simulink model "Station_1_Distributing_Testing"  (R2024a)
settings: Solver=FixedStepAuto  StartTime=0.0  StopTime=30  FixedStep=0.1  RelTol=1e-3
libraries: opcualib x1
settings Model: PacingRate=0.500000  Creator=admin  LastModifiedBy=admin

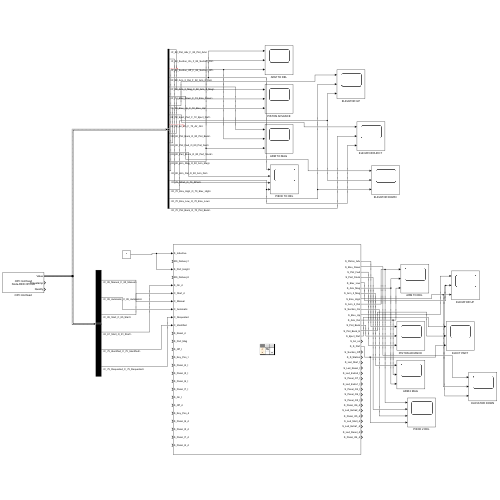
[thumbnail: Simulink's stored preview of the top-level diagram]
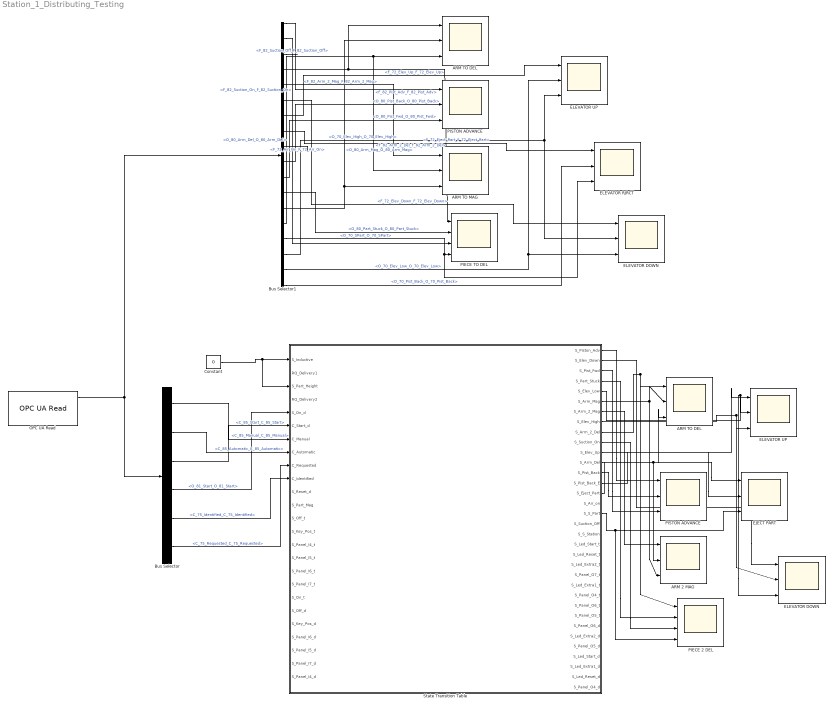
== system Station_1_Distributing_Testing ==
  "ARM 2 MAG " : Scope  NumInputPorts=3
  ARM TO DEL : Scope  NumInputPorts=3
  "ARM TO DEL " : Scope  NumInputPorts=3
  "ARM TO MAG " : Scope  NumInputPorts=3
  Bus Selector : BusSelector  OutputSignals=C_85_Manual_C_85_Manual,C_85_Automatic_C_85_Automatic,C_85_Start_C_85_Start,O_81_Start_O_81_Start,C_75_Identified_C_75_Identified,C_75_Requested_C_75_Requested
  Bus Selector1 : BusSelector  OutputSignals=F_82_Pist_Adv_F_82_Pist_Adv,F_82_Suction_On_F_82_Suction_On,F_82_Suction_Off_F_82_Suction_Off,F_82_Arm_2_Del_F_82_Arm_2_Del,F_82_Arm_2_Mag_F_82_Arm_2_Mag,F_72_Elev_Down_F_72_Elev_Down,F_72_Elev_Up_F_72_Elev_Up,F_72_Eject_Part_F_72_Eject_Part,F_72_Air_On_F_72_Air_On,O_80_Pist_Back_O_80_Pist_Back,O_80_Pist_Fwd_O_80_Pist_Fwd,O_80_Part_Stuck_O_80_Part_Stuck,O_80_Arm_Mag_O_80_Arm_Mag,O_80_Arm_Del_O_80_Arm_Del,O_70_SPart_O_70_SPart,O_70_Elev_High_O_70_Elev_High,O_70_Elev_Low_O_70_Elev_Low,O_70_Pist_Back_O_70_Pist_Back
  Constant : Constant  Value=0
  EJECT PART : Scope  NumInputPorts=3
  ELEVATOR DOWN : Scope  NumInputPorts=3
  "ELEVATOR DOWN " : Scope  NumInputPorts=3
  "ELEVATOR RJRCT " : Scope  NumInputPorts=3
  ELEVATOR UP : Scope  NumInputPorts=3
  "ELEVATOR UP " : Scope  NumInputPorts=3
  OPC UA Read : opcualib/OPC UA Read  SelectedServer=Node-RED OPCUA  ServerList=Node-RED OPCUA  NodeList={ '1', 'C_85_Manual', '17', 'C_85_Manual', '0'; '2', 'C_85_Automatic', '17', 'C_85_Automatic', '0'; '3', 'C_85_Start', '17', 'C_85_Start', '0'; '4', 'O_81_Start', '17', 'O_81_Start', '0'; '5', 'F_82_Pist_Adv', '17', 'F_82_Pist_Adv', '0'; '6', 'F_82_Suction_On', '17', 'F_82_Suction_On', '0'; '7', 'F_82_Suction_Off', '17', 'F_82_Suction_Off', '0'; '8', 'F_82_Arm_2_Del', '17', 'F_82_Arm_2_Del', '0'; '9', 'F_82_Arm_2_Mag', '17', 'F_82_Arm_2_Mag', '0'; '10', 'F_72_Elev_Down', '16', 'F_72_Elev_Down', '0'; '11', 'F_72_Elev_Up', '16', 'F_72_Elev_Up', '0'; '12', 'F_72_Eject_Part', '16', 'F_72_Eject_Part', '0'; '13', 'F_72_Air_On', '16', 'F_72_Air_On', '0'; '14', 'C_75_Identified', '16', 'C_75_Identified', '0'; '15', 'C_75_Requested', '16', 'C_75_Requested', '0'; '16', 'O_80_Pist_Back', '17', 'O_80_Pist_Back', '0'; '17', 'O_80_Pist_Fwd', '17', 'O_80_Pist_Fwd', '0'; '18', 'O_80_Part_Stuck', '17', 'O_80_Part_Stuck', '0'; '19', 'O_80_Arm_Mag', '17', 'O_80_Arm_Mag', '0'; '20', 'O_80_Arm_Del', '17', 'O_80_Arm_Del', '0'; '21', 'O_70_SPart', '16', 'O_70_SPart', '0'; '22', 'O_70_Elev_High', '16', 'O_70_Elev_High', '0'; '23', 'O_70_Elev_Low', '16', 'O_70_Elev_Low', '0'; '24', 'O_70_Pist_Back', '16', 'O_70_Pist_Back', '0' }  ShowQualityPort=on  ShowTimestampPort=on  ShowTimestampPortAs=Seconds since start  SampleTime=-1
  PIECE 2 DEL : Scope  NumInputPorts=4
  PIECE TO DEL : Scope  NumInputPorts=4
  PISTON ADVANCE : Scope  NumInputPorts=3
  "PISTON ADVANCE " : Scope  NumInputPorts=3
  State Transition Table : State Transition Table  TreatAsAtomicUnit=on
      settings: PortSchema="{\"entries\":[{\"content\":{\"sides\":[{\"content\":{\"connectorIds\":[\"In1\",\"In2\",\"In3\",\"In4\",\"In5\",\"In6\",\"In7\",\"In8\",\"In9\",\"In10\",\"In11\",\"In12\",\"In13\",\"In14\",\"In15\",\"In16\",\"In17\",\"In18\",\"In19\",\"In20\",\"In21\",\"In22\",\"In23\",\"In24\",\"In25\"]},\"type\":\"ConnectorPlacement.EquallySpacedRectSide\",\"uuid\":\"c1ffde1c-4698-47c1-b8e1-e37e2294cce5\"},{\"content\":{\"connectorIds\":[\"Out1\",\"Out2\",\"Out3\",\"Out4\",\"Out5\",\"Out6\",\"Out7\",\"Out8\",\"Out10\",\"Out9\",\"Out11\",\"Out12\",\"Out13\",\"Out14\",\"Out15\",\"Out16\",\"Out17\",\"Out18\",\"Out19\",\"Out20\",\"Out21\",\"Out22\",\"Out23\",\"Out24\",\"Out25\",\"Out26\",\"Out27\",\"Out28\",\"Out29\",\"Out30\",\"Out31\",\"Out32\",\"Out33\",\"Out34\"],\"side\":\"RIGHT\"},\"type\":\"ConnectorPlacement.EquallySpacedRectSide\",\"uuid\":\"c7cc1e75-ba3b-429d-be47-1a37eca50664\"},{\"content\":{\"side\":\"TOP\"},\"type\":\"ConnectorPlacement.EquallySpacedRectSide\",\"uuid\":\"a3e10976-981e-41c1-9e4c-ac87463bc268\"}]},\"type\":\"ConnectorPlacement.EquallySpacedConnector\",\"uuid\":\"49dd4243-5969-4559-99a9-f798051ededc\"}],\"packageUris\":[\"http://schema.mathworks.com/mf0/Connector/R2020b\"],\"version\":\"1.0\"}"
  wires:
  OPC UA Read/1 -> Bus Selector/1, Bus Selector1/1
  Bus Selector/1 -> State Transition Table/7(C_Manual)  "<C_85_Manual_C_85_Manual>"
  Bus Selector/2 -> State Transition Table/8(C_Automatic)  "<C_85_Automatic_C_85_Automatic>"
  Bus Selector/4 -> State Transition Table/5(S_On_d)  "<O_81_Start_O_81_Start>"
  Bus Selector/3 -> State Transition Table/6(C_Start_d)  "<C_85_Start_C_85_Start>"
  Constant/1 -> State Transition Table/1(S_Inductive), State Transition Table/3(S_Part_Height)
  Bus Selector/5 -> State Transition Table/10(C_Identified)  "<C_75_Identified_C_75_Identified>"
  Bus Selector/6 -> State Transition Table/9(C_Requested)  "<C_75_Requested_C_75_Requested>"
  Bus Selector1/1 -> PISTON ADVANCE/1  "<F_82_Pist_Adv_F_82_Pist_Adv>"
  Bus Selector1/2 -> PIECE TO DEL/3  "<F_82_Suction_On_F_82_Suction_On>"
  Bus Selector1/3 -> ?  "<F_82_Suction_Off_F_82_Suction_Off>"
  Bus Selector1/4 -> PIECE TO DEL/1, ARM TO DEL/1  "<F_82_Arm_2_Del_F_82_Arm_2_Del>"
  Bus Selector1/5 -> "ARM TO MAG "/1  "<F_82_Arm_2_Mag_F_82_Arm_2_Mag>"
  Bus Selector1/6 -> "ELEVATOR DOWN "/1  "<F_72_Elev_Down_F_72_Elev_Down>"
  Bus Selector1/7 -> ELEVATOR UP/1  "<F_72_Elev_Up_F_72_Elev_Up>"
  Bus Selector1/8 -> "ELEVATOR RJRCT "/1  "<F_72_Eject_Part_F_72_Eject_Part>"
  Bus Selector1/9 -> ?  "<F_72_Air_On_F_72_Air_On>"
  Bus Selector1/10 -> PISTON ADVANCE/2  "<O_80_Pist_Back_O_80_Pist_Back>"
  Bus Selector1/11 -> PISTON ADVANCE/3  "<O_80_Pist_Fwd_O_80_Pist_Fwd>"
  Bus Selector1/13 -> "ARM TO MAG "/3, ARM TO DEL/2  "<O_80_Arm_Mag_O_80_Arm_Mag>"
  Bus Selector1/14 -> ARM TO DEL/3, "ARM TO MAG "/2  "<O_80_Arm_Del_O_80_Arm_Del>"
  Bus Selector1/15 -> "ELEVATOR RJRCT "/3, PIECE TO DEL/4  "<O_70_SPart_O_70_SPart>"
  Bus Selector1/16 -> "ELEVATOR DOWN "/2, ELEVATOR UP/3  "<O_70_Elev_High_O_70_Elev_High>"
  Bus Selector1/17 -> "ELEVATOR DOWN "/3, ELEVATOR UP/2  "<O_70_Elev_Low_O_70_Elev_Low>"
  Bus Selector1/18 -> "ELEVATOR RJRCT "/2  "<O_70_Pist_Back_O_70_Pist_Back>"
  Bus Selector1/12 -> PIECE TO DEL/2  "<O_80_Part_Stuck_O_80_Part_Stuck>"
  State Transition Table/10(S_Arm_2_Del) -> PIECE 2 DEL/1, "ARM TO DEL "/1
  State Transition Table/6(S_Arm_Mag) -> "ARM 2 MAG "/3, "ARM TO DEL "/2
  State Transition Table/12(S_Arm_Del) -> "ARM 2 MAG "/2, "ARM TO DEL "/3
  State Transition Table/1(S_Piston_Adv) -> "PISTON ADVANCE "/1
  State Transition Table/13(S_Pist_Back) -> "PISTON ADVANCE "/2
  State Transition Table/3(S_Pist_Fwd) -> "PISTON ADVANCE "/3
  State Transition Table/7(S_Arm_2_Mag) -> "ARM 2 MAG "/1
  State Transition Table/4(S_Part_Stuck) -> PIECE 2 DEL/2
  State Transition Table/9(S_Suction_On) -> PIECE 2 DEL/3
  State Transition Table/11(S_Elev_Up) -> "ELEVATOR UP "/1
  State Transition Table/5(S_Elev_Low) -> ELEVATOR DOWN/3, "ELEVATOR UP "/2
  State Transition Table/8(S_Elev_High) -> ELEVATOR DOWN/2, "ELEVATOR UP "/3
  State Transition Table/15(S_Eject_Part) -> EJECT PART/1
  State Transition Table/14(S_Pist_Back_E) -> EJECT PART/2
  State Transition Table/17(S_S_Part) -> PIECE 2 DEL/4, EJECT PART/3
  State Transition Table/2(S_Elev_Down) -> ELEVATOR DOWN/1

== stateflow chart Station_1_Distributing_Testing/State Transition Table ==
  state state1
    S_Arm_2_Del=0;
    S_Arm_2_Mag=0;
    S_Piston_Adv=0;
    S_Elev_Up=0;
    S_Elev_Down=0;
    S_Eject_Part=0;
    S_Air_on=0;
    S_Suction_On=0;
    S_Suction_Off=0;
    S_Arm_Mag=1;
    S_Arm_Del=0;
    S_Part_Stuck=0;
    S_Pist_Fwd=0;
    S_Pist_Back=1;
    S_Elev_Low=1;
    S_Elev_High=0;
    S_S_Part=0;
    S_Pist_Back_E=1;
    S_S_Station=0;
    S_On_t;
    S_Off_t;
    S_Key_Pos_t;
    S_Panel_I4_t;
    S_Panel_I5_t;
    S_Panel_I6_t;
    S_Panel_I7_t;
    S_Led_Start_t=0;
    S_Led_Reset_t=0;
    S_Led_Extra1_t=0;
    S_Led_Extra2_t=0;
    S_Panel_O4_t=0;
    S_Panel_O5_t=0;
    S_Panel_O6_t=0;
    S_Panel_O7_t=0;
    S_Off_d;
    S_Key_Pos_d;
    S_Panel_I4_d;
    S_Panel_I5_d;
    S_Panel_I6_d;
    S_Panel_I7_d;
    S_Led_Start_d=0;
    S_Led_Reset_d=0;
    S_Led_Extra1_d=0;
    S_Led_Extra2_d=0;
    S_Panel_O4_d=0;
    S_Panel_O5_d=0;
    S_Panel_O6_d=0;
  state dis_cont_arm_to_del
    S_Arm_2_Del=1;
    S_Arm_2_Mag=0;
    S_Piston_Adv=0;
    S_Elev_Up=0;
    S_Elev_Down=0;
    S_Eject_Part=0;
    S_Air_on=0;
    S_Suction_On=0;
    state dis_cont_arm_to_del_1
    (default) -> dis_cont_arm_to_del_1
    dis_cont_arm_to_del_1 -> (junction 261) : after(0.73,sec)
        | {S_Arm_Mag=0;}
    (junction 261) -> dis_cont_arm_to_del_1
  state piston_advance
    S_Arm_2_Del=0;
    S_Arm_2_Mag=0;
    S_Piston_Adv=1;
    S_Elev_Up=0;
    S_Elev_Down=0;
    S_Eject_Part=0;
    S_Air_on=0;
    S_Suction_On=0;
    state piston_advance_1
    (default) -> piston_advance_1
    piston_advance_1 -> (junction 257) : {S_Pist_Back=0;
        | S_Pist_Fwd=1;}
    (junction 257) -> piston_advance_1
  state arm_to_mag
    S_Arm_2_Del=0;
    S_Arm_2_Mag=1;
    S_Piston_Adv=0;
    S_Elev_Up=0;
    S_Elev_Down=0;
    S_Eject_Part=0;
    S_Air_on=0;
    S_Suction_On=0;
    state arm_to_mag_1
    (default) -> arm_to_mag_1
    arm_to_mag_1 -> (junction 269) : after(0.5,sec)
        | {S_Arm_Del=0;}
    (junction 269) -> arm_to_mag_1
  state arm_with_piece_to_del
    S_Arm_2_Del=1;
    S_Arm_2_Mag=0;
    S_Piston_Adv=0;
    S_Elev_Up=0;
    S_Elev_Down=0;
    S_Eject_Part=0;
    S_Air_on=0;
    S_Suction_On=1;
    state arm_with_piece_to_del_1
    (default) -> arm_with_piece_to_del_1
    arm_with_piece_to_del_1 -> (junction 265) : after(0.73,sec)
        | {S_Arm_Mag=0;}
    (junction 265) -> arm_with_piece_to_del_1
  state arm_to_mag1
    S_Arm_2_Del=0;
    S_Arm_2_Mag=1;
    S_Piston_Adv=0;
    S_Elev_Up=0;
    S_Elev_Down=0;
    S_Eject_Part=0;
    S_Air_on=0;
    S_Suction_On=0;
    state arm_to_mag1_1
    state arm_to_mag1_2
    arm_to_mag1_2 -> (junction 974) : after(0.2,sec)
        | {S_Arm_Del=0;}
    (default) -> arm_to_mag1_1
    arm_to_mag1_1 -> arm_to_mag1_2 : [after(0.5,sec)]
        | {S_Suction_Off=0;}
    (junction 974) -> arm_to_mag1_2
  state elevator_up
    S_Arm_2_Del=0;
    S_Arm_2_Mag=0;
    S_Piston_Adv=0;
    S_Elev_Up=1;
    S_Elev_Down=0;
    S_Eject_Part=0;
    S_Air_on=0;
    S_Suction_On=0;
    state elevator_up_1
    state elevator_up_2
    state elevator_up_3
    state elevator_up_4
    elevator_up_4 -> (junction 1045) : after(0.65,sec)
        | {S_Elev_High=1;}
    (default) -> elevator_up_1
    elevator_up_1 -> elevator_up_2 : after(0.5,sec)
        | {S_Elev_Low=0;}
    elevator_up_2 -> elevator_up_3 : after(0.1,sec)
        | {S_S_Station=1;}
    elevator_up_3 -> elevator_up_4 : after(0.3,sec)
        | {S_S_Station=1;}
    (junction 1045) -> elevator_up_4
  state decision
  state accepted
    S_Arm_2_Del=0;
    S_Arm_2_Mag=0;
    S_Piston_Adv=0;
    S_Elev_Up=1;
    S_Elev_Down=0;
    S_Eject_Part=1;
    S_Air_on=1;
    S_Suction_On=0;
    state accepted_1
    (default) -> accepted_1
    accepted_1 -> (junction 291) : after(0.2,sec)
        | {S_Pist_Back_E=0;}
    (junction 291) -> accepted_1
  state elevator_down
    S_Arm_2_Del=0;
    S_Arm_2_Mag=0;
    S_Piston_Adv=0;
    S_Elev_Up=0;
    S_Elev_Down=1;
    S_Eject_Part=0;
    S_Air_on=1;
    S_Suction_On=0;
    state elevator_down_1
    state elevator_down_2
    state elevator_down_3
    state elevator_down_4
    elevator_down_4 -> (junction 987) : after(0.3,sec)
        | {S_S_Station=0;}
    (default) -> elevator_down_1
    elevator_down_1 -> elevator_down_2 : after(0.2,sec)
        | {S_Pist_Back_E=1;}
    elevator_down_2 -> elevator_down_3 : after(0.1,sec)
        | {S_Elev_High=0;}
    elevator_down_3 -> elevator_down_4 : after(0.7,sec)
        | {S_S_Station=1;}
    (junction 987) -> elevator_down_4
  state elev_is_down_but_air
    S_Arm_2_Del=0;
    S_Arm_2_Mag=0;
    S_Piston_Adv=0;
    S_Elev_Up=0;
    S_Elev_Down=0;
    S_Eject_Part=0;
    S_Air_on=1;
    S_Suction_On=0;
  state rejected
    S_Arm_2_Del=0;
    S_Arm_2_Mag=0;
    S_Piston_Adv=0;
    S_Elev_Up=0;
    S_Elev_Down=1;
    S_Eject_Part=0;
    S_Air_on=0;
    S_Suction_On=0;
    state rejected_1
    state rejected_2
    state rejected_3
    rejected_3 -> (junction 993) : after(0.3,sec)
        | {S_S_Station=0;}
    (default) -> rejected_1
    rejected_1 -> rejected_2 : after(0.3,sec)
        | {S_Elev_High=0;}
    rejected_2 -> rejected_3 : after(0.7,sec)
        | {S_S_Station=1;}
    (junction 993) -> rejected_3
  state rejection_ejection
    S_Arm_2_Del=0;
    S_Arm_2_Mag=0;
    S_Piston_Adv=0;
    S_Elev_Up=0;
    S_Elev_Down=0;
    S_Eject_Part=1;
    S_Air_on=0;
    S_Suction_On=0;
    state rejection_ejection_1
    (default) -> rejection_ejection_1
    rejection_ejection_1 -> (junction 305) : after(0.2,sec)
        | {S_Pist_Back_E=0;}
    (junction 305) -> rejection_ejection_1
  state pistonback
  state cont_arm_to_delivery
    S_Arm_2_Del=1;
    S_Arm_2_Mag=0;
    S_Piston_Adv=0;
    S_Elev_Up=0;
    S_Elev_Down=0;
    S_Eject_Part=0;
    S_Air_on=0;
    S_Suction_On=0;
    state cont_arm_to_delivery_1
    (default) -> cont_arm_to_delivery_1
    cont_arm_to_delivery_1 -> (junction 317) : after(0.73,sec)
        | {S_Arm_Mag=0;}
    (junction 317) -> cont_arm_to_delivery_1
  state arm_to_delivery_pist_adv
    S_Arm_2_Del=1;
    S_Arm_2_Mag=0;
    S_Piston_Adv=1;
    S_Elev_Up=0;
    S_Elev_Down=0;
    S_Eject_Part=0;
    S_Air_on=0;
    S_Suction_On=0;
    state arm_to_delivery_pist_adv_1
    (default) -> arm_to_delivery_pist_adv_1
    arm_to_delivery_pist_adv_1 -> (junction 555) : {S_Pist_Fwd=1;
        | S_Pist_Back=0;}
    (junction 555) -> arm_to_delivery_pist_adv_1
  state arm_to_mag_cont
    S_Arm_2_Del=0;
    S_Arm_2_Mag=1;
    S_Piston_Adv=0;
    S_Elev_Up=0;
    S_Elev_Down=0;
    S_Eject_Part=0;
    S_Air_on=0;
    S_Suction_On=0;
    state arm_to_mag_cont_1
    (default) -> arm_to_mag_cont_1
    arm_to_mag_cont_1 -> (junction 324) : after(0.73,sec)
        | {S_Arm_Del=0;}
    (junction 324) -> arm_to_mag_cont_1
  state piece_to_del1
    S_Arm_2_Del=1;
    S_Arm_2_Mag=0;
    S_Piston_Adv=0;
    S_Elev_Up=0;
    S_Elev_Down=0;
    S_Eject_Part=0;
    S_Air_on=0;
    S_Suction_On=1;
    state piece_to_del1_1
    (default) -> piece_to_del1_1
    piece_to_del1_1 -> (junction 396) : after(0.73,sec)
        | {S_Arm_Mag=0;}
    (junction 396) -> piece_to_del1_1
  state piece_to_del2
    S_Arm_2_Del=1;
    S_Arm_2_Mag=0;
    S_Piston_Adv=0;
    S_Elev_Up=0;
    S_Elev_Down=0;
    S_Eject_Part=0;
    S_Air_on=0;
    S_Suction_On=1;
  state arm_to_mag_pist_adv
    S_Arm_2_Del=0;
    S_Arm_2_Mag=1;
    S_Piston_Adv=1;
    S_Elev_Up=0;
    S_Elev_Down=0;
    S_Eject_Part=0;
    S_Air_on=0;
    S_Suction_On=0;
    state arm_to_mag_pist_adv_1
    state arm_to_mag_pist_adv_2
    arm_to_mag_pist_adv_2 -> (junction 997) : after(0.3,sec)
        | {S_Suction_Off=0;}
    (default) -> arm_to_mag_pist_adv_1
    arm_to_mag_pist_adv_1 -> arm_to_mag_pist_adv_2 : after(0.2,sec)
        | {S_S_Part=1;}
    (junction 997) -> arm_to_mag_pist_adv_2
  state rest_of_arm_to_mag
    S_Arm_2_Del=0;
    S_Arm_2_Mag=1;
    S_Piston_Adv=0;
    S_Elev_Up=0;
    S_Elev_Down=0;
    S_Eject_Part=0;
    S_Air_on=0;
    S_Suction_On=0;
    state rest_of_arm_to_mag_1
    (default) -> rest_of_arm_to_mag_1
    rest_of_arm_to_mag_1 -> (junction 410) : after(0.13,sec)
        | {S_Arm_Del=0;}
    (junction 410) -> rest_of_arm_to_mag_1
  state elevtor_up_cont
    S_Arm_2_Del=0;
    S_Arm_2_Mag=0;
    S_Piston_Adv=0;
    S_Elev_Up=1;
    S_Elev_Down=0;
    S_Eject_Part=0;
    S_Air_on=0;
    S_Suction_On=1;
    S_Part_Stuck=1;
    state elevtor_up_cont_1
    state elevtor_up_cont_2
    state elevtor_up_cont_3
    state elevtor_up_cont_4
    elevtor_up_cont_4 -> (junction 1005) : after(0.65,sec)
        | {S_Elev_High=1;}
    (default) -> elevtor_up_cont_1
    elevtor_up_cont_1 -> elevtor_up_cont_2 : after(0.50,sec)
        | {S_Elev_Low=0;}
    elevtor_up_cont_2 -> elevtor_up_cont_3 : after(0.1,sec)
        | {S_S_Station=1;}
    elevtor_up_cont_3 -> elevtor_up_cont_4 : after(0.3,sec)
        | {S_S_Station=0;}
    (junction 1005) -> elevtor_up_cont_4
  state decicion_2
  state accept2
    S_Arm_2_Del=0;
    S_Arm_2_Mag=0;
    S_Piston_Adv=0;
    S_Elev_Up=1;
    S_Elev_Down=0;
    S_Eject_Part=1;
    S_Air_on=1;
    S_Suction_On=1;
    state accept2_1
    (default) -> accept2_1
    accept2_1 -> (junction 571) : after(0.2,sec)
        | {S_Pist_Back_E=0;}
    (junction 571) -> accept2_1
  state elevator_down2
    S_Arm_2_Del=0;
    S_Arm_2_Mag=0;
    S_Piston_Adv=0;
    S_Elev_Up=0;
    S_Elev_Down=1;
    S_Eject_Part=0;
    S_Air_on=1;
    S_Suction_On=1;
    state elevator_down2_1
      state elevator_down2_1_1
        state elevator_down2_1_1_1
        (default) -> elevator_down2_1_1_1
        elevator_down2_1_1_1 -> (junction 848) : after(0.3,sec)
            | {S_Elev_High=0;}
        (junction 848) -> elevator_down2_1_1_1
      (default) -> elevator_down2_1_1
      elevator_down2_1_1 -> (junction 443) : after(1,sec)
          | {S_S_Station=1;}
      (junction 443) -> elevator_down2_1_1
    (default) -> elevator_down2_1
    elevator_down2_1 -> (junction 439) : after(1.3,sec)
        | {S_S_Station=0;}
    (junction 439) -> elevator_down2_1
  state to_del2_1
    S_Arm_2_Del=1;
    S_Arm_2_Mag=0;
    S_Piston_Adv=0;
    S_Elev_Up=0;
    S_Elev_Down=0;
    S_Eject_Part=0;
    S_Air_on=1;
    S_Suction_On=1;
    state to_del2_1_1
    (default) -> to_del2_1_1
    to_del2_1_1 -> (junction 575) : after(0.73,sec)
        | {S_Arm_Mag=0;}
    (junction 575) -> to_del2_1_1
  state reject2
    S_Arm_2_Del=0;
    S_Arm_2_Mag=0;
    S_Piston_Adv=0;
    S_Elev_Up=0;
    S_Elev_Down=1;
    S_Eject_Part=0;
    S_Air_on=0;
    S_Suction_On=1;
    state reject2_1
    state reject2_2
    state reject2_3
    reject2_3 -> (junction 1012) : after(0.3,sec)
        | {S_S_Station=0;}
    (default) -> reject2_1
    reject2_1 -> reject2_2 : after(0.3,sec)
        | {S_Elev_High=0;}
    reject2_2 -> reject2_3 : after(0.7,sec)
        | {S_S_Station=1;}
    (junction 1012) -> reject2_3
  state arm_to_del_with_eject
    S_Arm_2_Del=1;
    S_Arm_2_Mag=0;
    S_Piston_Adv=0;
    S_Elev_Up=0;
    S_Elev_Down=0;
    S_Eject_Part=1;
    S_Air_on=0;
    S_Suction_On=1;
    state arm_to_del_with_eject_1
    state arm_to_del_with_eject_2
    arm_to_del_with_eject_2 -> (junction 1020) : after(0.5,sec)
        | {S_Arm_Mag=0;}
    (default) -> arm_to_del_with_eject_1
    arm_to_del_with_eject_1 -> arm_to_del_with_eject_2 : after(0.2,sec)
        | {S_Pist_Back_E=0;}
    (junction 1020) -> arm_to_del_with_eject_2
  state after_last_piece_delivery
    S_Arm_2_Del=0;
    S_Arm_2_Mag=1;
    S_Piston_Adv=0;
    S_Elev_Up=0;
    S_Elev_Down=0;
    S_Eject_Part=0;
    S_Air_on=0;
    S_Suction_On=0;
    state after_last_piece_delivery_1
    state after_last_piece_delivery_2
    after_last_piece_delivery_2 -> (junction 1016) : after(0.50,sec)
        | {S_Arm_Del=0;}
    (default) -> after_last_piece_delivery_1
    after_last_piece_delivery_1 -> after_last_piece_delivery_2 : after(0.2,sec)
        | {S_S_Part=1;}
    (junction 1016) -> after_last_piece_delivery_2
  state elevator_up_with_to_mag
    S_Arm_2_Del=0;
    S_Arm_2_Mag=1;
    S_Piston_Adv=0;
    S_Elev_Up=1;
    S_Elev_Down=0;
    S_Eject_Part=0;
    S_Air_on=0;
    S_Suction_On=0;
  state elevator_up_only
    S_Arm_2_Del=0;
    S_Arm_2_Mag=1;
    S_Piston_Adv=0;
    S_Elev_Up=1;
    S_Elev_Down=0;
    S_Eject_Part=0;
    S_Air_on=0;
    S_Suction_On=0;
    state elevator_up_only_1
    state elevator_up_only_2
    state elevator_up_only_3
    state elevator_up_only_4
    elevator_up_only_4 -> (junction 1028) : after(0.65,sec)
        | {S_Elev_High=1;}
    (default) -> elevator_up_only_1
    elevator_up_only_1 -> elevator_up_only_2 : after(0.3,sec)
        | {S_Elev_Low=0;}
    elevator_up_only_2 -> elevator_up_only_3 : after(0.1,sec)
        | {S_S_Station=1;}
    elevator_up_only_3 -> elevator_up_only_4 : after(0.3,sec)
        | {S_S_Station=0;}
    (junction 1028) -> elevator_up_only_4
  state decision_3
  state accept
    S_Arm_2_Del=0;
    S_Arm_2_Mag=0;
    S_Piston_Adv=0;
    S_Elev_Up=1;
    S_Elev_Down=0;
    S_Eject_Part=1;
    S_Air_on=1;
    S_Suction_On=0;
  state elev_down_4
    S_Arm_2_Del=0;
    S_Arm_2_Mag=0;
    S_Piston_Adv=0;
    S_Elev_Up=0;
    S_Elev_Down=1;
    S_Eject_Part=0;
    S_Air_on=1;
    S_Suction_On=0;
    state elev_down_4_1
    state elev_down_4_2
    state elev_down_4_3
    state elev_down_4_4
    elev_down_4_4 -> (junction 1036) : after(0.3,sec)
        | {S_S_Station=0;}
    (default) -> elev_down_4_1
    elev_down_4_1 -> elev_down_4_2 : after(0.2,sec)
        | {S_Pist_Back_E=1;}
    elev_down_4_2 -> elev_down_4_3 : after(0.1,sec)
        | {S_Elev_High=0;}
    elev_down_4_3 -> elev_down_4_4 : after(0.7,sec)
        | {S_S_Station=1;}
    (junction 1036) -> elev_down_4_4
  state air_still_on
    S_Arm_2_Del=0;
    S_Arm_2_Mag=0;
    S_Piston_Adv=0;
    S_Elev_Up=0;
    S_Elev_Down=0;
    S_Eject_Part=0;
    S_Air_on=1;
    S_Suction_On=0;
  state reject_elev_down
    S_Arm_2_Del=0;
    S_Arm_2_Mag=0;
    S_Piston_Adv=0;
    S_Elev_Up=0;
    S_Elev_Down=1;
    S_Eject_Part=0;
    S_Air_on=0;
    S_Suction_On=0;
    state reject_elev_down_1
    state reject_elev_down_2
    state reject_elev_down_3
    reject_elev_down_3 -> (junction 1042) : after(0.3,sec)
        | {S_S_Station=0;}
    (default) -> reject_elev_down_1
    reject_elev_down_1 -> reject_elev_down_2 : after(0.3,sec)
        | {S_Elev_High=0;}
    reject_elev_down_2 -> reject_elev_down_3 : after(0.7,sec)
        | {S_S_Station=1;}
    (junction 1042) -> reject_elev_down_3
  state ejecting_part
    S_Arm_2_Del=0;
    S_Arm_2_Mag=0;
    S_Piston_Adv=0;
    S_Elev_Up=0;
    S_Elev_Down=0;
    S_Eject_Part=1;
    S_Air_on=0;
    S_Suction_On=0;
    state ejecting_part_1
    (default) -> ejecting_part_1
    ejecting_part_1 -> (junction 583) : after(0.2,sec)
        | {S_Pist_Back_E=0;}
    (junction 583) -> ejecting_part_1
  state piston_back_sensor
  state RESET
    S_Arm_2_Del=0;
    S_Arm_2_Mag=0;
    S_Piston_Adv=0;
    S_Elev_Up=0;
    S_Elev_Down=0;
    S_Eject_Part=0;
    S_Air_on=0;
    S_Suction_On=0;
    S_Suction_Off=0;
  state reset_RETURN_ARM_TO_MAG_with_suction
    S_Arm_2_Del=0;
    S_Arm_2_Mag=1;
    S_Piston_Adv=0;
    S_Elev_Up=0;
    S_Elev_Down=0;
    S_Eject_Part=0;
    S_Air_on=0;
    S_Suction_On=1;
    S_Suction_Off=0;
  state suction_off_reset
    S_Arm_2_Del=0;
    S_Arm_2_Mag=0;
    S_Piston_Adv=0;
    S_Elev_Up=0;
    S_Elev_Down=0;
    S_Eject_Part=0;
    S_Air_on=0;
    S_Suction_On=0;
    S_Suction_Off=1;
  state reset_return_arm_to_mag
    S_Arm_2_Del=0;
    S_Arm_2_Mag=1;
    S_Piston_Adv=0;
    S_Elev_Up=0;
    S_Elev_Down=0;
    S_Eject_Part=0;
    S_Air_on=0;
    S_Suction_On=0;
    S_Suction_Off=0;
  (default) -> state1
  (junction 207) -> state1
  state1 -> (junction 68) [order 2] : [((S_On_d==1 || C_Start_d==1) && (C_Manual==0 && C_Automatic==1))&& S_Part_Mag==0 ]
  (junction 209) -> (junction 207)
  (junction 68) -> (junction 66)
  state1 -> dis_cont_arm_to_del [order 1] : [((S_On_d==1 ||C_Start_d==1 )&& (C_Manual==1 && C_Automatic==0))&&S_Part_Mag==0 ]
  dis_cont_arm_to_del -> (junction 626) [order 2] : [S_Reset_d==1]
      | {S_Led_Reset_d=1;}
  (junction 626) -> (junction 629)
  dis_cont_arm_to_del -> piston_advance [order 1] : after(1.55,sec)
      | {S_Arm_Del=1;}
  piston_advance -> (junction 629) [order 2] : [S_Reset_d==1]
      | {S_Led_Reset_d=1;}
  (junction 629) -> (junction 632)
  piston_advance -> arm_to_mag [order 1] : after(0.6,sec)
      | {S_Pist_Back=1;
      | S_Pist_Fwd=0;}
  arm_to_mag -> (junction 632) [order 2] : [S_Reset_d==1]
      | {S_Led_Reset_d=1;}
  (junction 632) -> (junction 635)
  arm_to_mag -> arm_with_piece_to_del [order 1] : after(0.9,sec)
      | {S_Arm_Mag=1;
      | S_Part_Stuck=1;}
  arm_with_piece_to_del -> (junction 635) [order 2] : [S_Reset_d==1]
      | {S_Led_Reset_d=1;}
  (junction 635) -> (junction 638)
  arm_with_piece_to_del -> arm_to_mag1 [order 1] : [after(1.525,sec)]
      | {S_Arm_Del=1;
      | S_Part_Stuck=0;
      | S_Suction_Off=1
      | S_S_Part=1;}
  arm_to_mag1 -> (junction 638) [order 3] : [S_Reset_d==1]
      | {S_Led_Reset_d=1;}
  (junction 638) -> (junction 641)
  arm_to_mag1 -> elevator_up [order 1] : [after(0.9,sec)&& S_Inductive==1]
      | {ID_Delivery1=0;
      | ID_Delivery2=1;
      | S_Arm_Mag=1;}
  arm_to_mag1 -> elevator_up [order 2] : [after(0.9,sec)&& S_Inductive==0]
      | {ID_Delivery1=1;
      | S_Arm_Mag=1;}
  (junction 775) -> elevator_up
  elevator_up -> (junction 641) [order 3] : [S_Reset_d==1]
      | {S_Led_Reset_d=1;}
  (junction 777) -> (junction 775)
  (junction 641) -> (junction 644)
  elevator_up -> decision [order 1] : [after(2,sec) && S_Part_Height==1]
      | {ID_Delivery2=1;}
  elevator_up -> decision [order 2] : [after(2,sec)&& S_Part_Height==0]
      | {ID_Delivery2=0;}
  decision -> (junction 43) [order 2] : [(C_Identified==0 &&C_Requested==1) && ((RQ_Delivery1~=ID_Delivery1) || (RQ_Delivery2~= ID_Delivery2))]
  (junction 43) -> (junction 41)
  decision -> (junction 644) [order 3] : [S_Reset_d==1]
      | {S_Led_Reset_d=1;}
  (junction 644) -> (junction 647)
  decision -> accepted [order 1] : [(C_Identified==1 && C_Requested==0)|| ((C_Identified==0 &&C_Requested==1) && RQ_Delivery1==ID_Delivery1&&RQ_Delivery2==ID_Delivery2)]
      | {S_S_Part=0;}
  accepted -> (junction 647) [order 2] : [S_Reset_d==1]
      | {S_Led_Reset_d=1;}
  (junction 647) -> (junction 650)
  accepted -> elevator_down [order 1] : after(1.2,sec)
  (junction 783) -> elevator_down
  elevator_down -> (junction 650) [order 2] : [S_Reset_d==1]
      | {S_Led_Reset_d=1;}
  (junction 785) -> (junction 783)
  (junction 650) -> (junction 653)
  elevator_down -> elev_is_down_but_air [order 1] : after(1.4,sec)
      | {S_Elev_Low=1;}
  elev_is_down_but_air -> (junction 209) [order 1] : after(1,sec)
  elev_is_down_but_air -> (junction 653) [order 2] : [S_Reset_d==1]
      | {S_Led_Reset_d=1;}
  (junction 311) -> (junction 209)
  (junction 653) -> (junction 656)
  (junction 41) -> rejected
  (junction 780) -> (junction 41)
  rejected -> (junction 656) [order 2] : [S_Reset_d==1]
      | {S_Led_Reset_d=1;}
  (junction 656) -> (junction 659)
  rejected -> rejection_ejection [order 1] : after(1.4,sec)
      | {S_Elev_Low=1;
      | S_S_Part=0;}
  rejection_ejection -> (junction 659) [order 2] : [S_Reset_d==1]
      | {S_Led_Reset_d=1;}
  (junction 659) -> (junction 662)
  rejection_ejection -> pistonback [order 1] : after(1,sec)
  pistonback -> (junction 311) [order 1] : after(0.2,sec)
      | {S_Pist_Back_E=1;}
  pistonback -> (junction 662) [order 2] : [S_Reset_d==1]
      | {S_Led_Reset_d=1;}
  (junction 222) -> (junction 311)
  (junction 662) -> (junction 665)
  (junction 66) -> cont_arm_to_delivery
  cont_arm_to_delivery -> (junction 665) [order 2] : [S_Reset_d==1]
  (junction 665) -> (junction 668)
  cont_arm_to_delivery -> arm_to_delivery_pist_adv [order 1] : after(1.5,sec)
  arm_to_delivery_pist_adv -> (junction 668) [order 2] : [S_Reset_d==1]
      | {S_Led_Reset_d=1;}
  (junction 668) -> (junction 671)
  arm_to_delivery_pist_adv -> arm_to_mag_cont [order 1] : after(0.6,sec)
      | {S_Arm_Del=1;
      | S_Pist_Back=1;
      | S_Pist_Fwd=0;}
  arm_to_mag_cont -> (junction 671) [order 2] : [S_Reset_d==1]
      | {S_Led_Reset_d=1;}
  (junction 671) -> (junction 674)
  arm_to_mag_cont -> piece_to_del1 [order 1] : after(0.9,sec)
      | {S_Arm_Mag=1;
      | S_Part_Stuck=1;}
  piece_to_del1 -> (junction 674) [order 2] : [S_Reset_d==1]
      | {S_Led_Reset_d=1;}
  (junction 674) -> (junction 677)
  piece_to_del1 -> piece_to_del2 [order 1] : [after(0.9,sec)]
      | {S_Suction_Off=1;}
  (junction 125) -> piece_to_del2
  piece_to_del2 -> (junction 144) [order 2] : [after(0.6,sec)&&S_Part_Mag==1]
  (junction 127) -> (junction 125)
  (junction 144) -> (junction 142)
  piece_to_del2 -> (junction 677) [order 3] : [S_Reset_d==1]
      | {S_Led_Reset_d=1;}
  (junction 677) -> (junction 680)
  piece_to_del2 -> arm_to_mag_pist_adv [order 1] : [after(0.6,sec)&&S_Part_Mag==0]
      | {S_Arm_Del=1;
      | S_Part_Stuck=0;
      | S_Suction_Off=1;
      | S_Pist_Fwd=1;
      | S_Pist_Back=0;}
  arm_to_mag_pist_adv -> (junction 680) [order 2] : [S_Reset_d==1]
      | {S_Led_Reset_d=1;}
  (junction 680) -> (junction 683)
  arm_to_mag_pist_adv -> rest_of_arm_to_mag [order 1] : [after(0.6,sec)]
      |
      | {S_Pist_Fwd=0;
      | S_Pist_Back=1;}
  rest_of_arm_to_mag -> (junction 683) [order 3] : [S_Reset_d==1]
      | {S_Led_Reset_d=1;}
  (junction 683) -> (junction 686)
  rest_of_arm_to_mag -> elevtor_up_cont [order 1] : [after(0.6,sec)&& S_Inductive==1]
      | {ID_Delivery1=0;
      | ID_Delivery2=1;
      | S_Arm_Mag=1;}
  rest_of_arm_to_mag -> elevtor_up_cont [order 2] : [after(0.6,sec)&& S_Inductive==0]
      | {ID_Delivery1=1;
      | S_Arm_Mag=1;}
  elevtor_up_cont -> (junction 686) [order 3] : [S_Reset_d==1]
      | {S_Led_Reset_d=1;}
  (junction 686) -> (junction 689)
  elevtor_up_cont -> decicion_2 [order 1] : [after(2,sec)&& S_Part_Height==1]
      | {ID_Delivery2=1;}
  elevtor_up_cont -> decicion_2 [order 2] : [after(2,sec)&& S_Part_Height==0]
      | {ID_Delivery2=0;}
  decicion_2 -> (junction 133) [order 2] : [(C_Identified==0 &&C_Requested==1)&& ((RQ_Delivery1~=ID_Delivery1) || (RQ_Delivery2~= ID_Delivery2))]
  (junction 133) -> (junction 131)
  decicion_2 -> (junction 689) [order 3] : [S_Reset_d==1]
      | {S_Led_Reset_d=1;}
  (junction 689) -> (junction 692)
  decicion_2 -> accept2 [order 1] : [(C_Identified==1 &&C_Requested==0)|| ((C_Identified==0 &&C_Requested==1)&&RQ_Delivery1==ID_Delivery1&&RQ_Delivery2==ID_Delivery2)]
      | {S_S_Part=0;}
  accept2 -> (junction 692) [order 2] : [S_Reset_d==1]
  (junction 692) -> (junction 695)
  accept2 -> elevator_down2 [order 1] : after(1,sec)
      | {S_Pist_Back_E=1;}
  elevator_down2 -> (junction 695) [order 2] : [S_Reset_d==1]
      | {S_Led_Reset_d=1;}
  (junction 695) -> (junction 698)
  elevator_down2 -> to_del2_1 [order 1] : after(1.5,sec)
      | {S_Elev_Low=1;}
  to_del2_1 -> (junction 127) [order 1] : after(0.9,sec)
      | {S_Arm_Del=1;}
  to_del2_1 -> (junction 698) [order 2] : [S_Reset_d==1]
      | {S_Led_Reset_d=1;}
  (junction 138) -> (junction 127)
  (junction 698) -> (junction 701)
  (junction 131) -> reject2
  reject2 -> (junction 701) [order 2] : [S_Reset_d==1]
      | {S_Led_Reset_d=1;}
  (junction 701) -> (junction 704)
  reject2 -> arm_to_del_with_eject [order 1] : after(1.5,sec)
      | {S_Elev_Low=1;
      | S_S_Part=0;}
  arm_to_del_with_eject -> (junction 138) [order 1] : after(0.9,sec)
      | {S_Arm_Del=1;
      | S_Part_Stuck=0;}
  arm_to_del_with_eject -> (junction 704) [order 2] : [S_Reset_d==1]
      | {S_Led_Reset_d=1;}
  (junction 704) -> (junction 707)
  (junction 142) -> after_last_piece_delivery
  after_last_piece_delivery -> (junction 707) [order 3] : [S_Reset_d==1]
      | {S_Led_Reset_d=1;}
  (junction 707) -> (junction 710)
  after_last_piece_delivery -> elevator_up_with_to_mag [order 1] : [after(1,sec)&& S_Inductive==1]
      | {ID_Delivery1=0;
      | ID_Delivery2=1;}
  after_last_piece_delivery -> elevator_up_with_to_mag [order 2] : [after(1,sec) && S_Inductive==0]
      | {ID_Delivery1=1;}
  elevator_up_with_to_mag -> (junction 710) [order 2] : [S_Reset_d==1]
      | {S_Led_Reset_d=1;}
  (junction 710) -> (junction 713)
  elevator_up_with_to_mag -> elevator_up_only [order 1] : [after(0.2,sec)]
      | {S_Arm_Mag=1;}
  elevator_up_only -> (junction 713) [order 3] : [S_Reset_d==1]
      | {S_Led_Reset_d=1;}
  (junction 713) -> (junction 716)
  elevator_up_only -> decision_3 [order 1] : [after(1.8,sec)&& S_Part_Height==1]
      | {ID_Delivery2=1;}
  elevator_up_only -> decision_3 [order 2] : [after(1.8,sec)&& S_Part_Height==0]
      | {ID_Delivery2=0;}
  decision_3 -> (junction 160) [order 2] : [(C_Identified==0 &&C_Requested==1) && ((RQ_Delivery1~=ID_Delivery1) || (RQ_Delivery2~= ID_Delivery2))]
  (junction 160) -> (junction 158)
  decision_3 -> (junction 716) [order 3] : [S_Reset_d==1]
      | {S_Led_Reset_d=1;}
  (junction 716) -> (junction 719)
  decision_3 -> accept [order 1] : [(C_Identified==1 && C_Requested==0) || ((C_Identified==0 &&C_Requested==1)&&RQ_Delivery1==ID_Delivery1&&RQ_Delivery2==ID_Delivery2)]
      | {S_S_Part=0;
      | S_Pist_Back_E=0;}
  accept -> (junction 719) [order 2] : [S_Reset_d==1]
      | {S_Led_Reset_d=1;}
  (junction 719) -> (junction 722)
  accept -> elev_down_4 [order 1] : after(1,sec)
  elev_down_4 -> (junction 722) [order 2] : [S_Reset_d==1]
      | {S_Led_Reset_d=1;}
  (junction 722) -> (junction 725)
  elev_down_4 -> air_still_on [order 1] : after(1.5,sec)
      | {S_Elev_Low=1;}
  air_still_on -> (junction 222) [order 1] : after(0.5,sec)
  air_still_on -> (junction 725) [order 2] : [S_Reset_d==1]
      | {S_Led_Reset_d=1;}
  (junction 540) -> (junction 222)
  (junction 725) -> (junction 728)
  (junction 158) -> reject_elev_down
  reject_elev_down -> (junction 728) [order 2] : [S_Reset_d==1]
      | {S_Led_Reset_d=1;}
  (junction 728) -> (junction 731)
  reject_elev_down -> ejecting_part [order 1] : after(1.5,sec)
      | {S_Elev_Low=1;
      | S_S_Part=0;}
  ejecting_part -> (junction 731) [order 2] : [S_Reset_d==1]
      | {S_Led_Reset_d=1;}
  (junction 731) -> (junction 624)
  ejecting_part -> piston_back_sensor [order 1] : after(1,sec)
  piston_back_sensor -> (junction 540) [order 1] : after(0.2,sec)
      | {S_Pist_Back_E=1;}
  (junction 744) -> (junction 540)
  piston_back_sensor -> RESET [order 2] : [S_Reset_d==1]
      | {S_Led_Reset_d=1;}
  RESET -> (junction 777) [order 3] : [S_Elev_Up==1|| S_S_Part==1]
  (junction 624) -> RESET
  RESET -> (junction 785) [order 5] : [S_Elev_Down==1 && S_S_Part==0]
  RESET -> (junction 751) [order 2] : [S_Arm_Mag==0 && S_Suction_On==0 && S_S_Part==0]
      | {S_Arm_Del=0;}
  (junction 751) -> (junction 749)
  RESET -> (junction 780) [order 4] : [S_Elev_Down==1 && S_S_Part==1]
  RESET -> reset_RETURN_ARM_TO_MAG_with_suction [order 1] : [S_Arm_Mag==0 && S_Suction_On==1 &&S_S_Part==0]
      | {S_Arm_Del=0;}
  reset_RETURN_ARM_TO_MAG_with_suction -> suction_off_reset : after(0.9,sec)
  suction_off_reset -> (junction 744) : after(0.5,sec)
  (junction 755) -> (junction 744)
  reset_return_arm_to_mag -> (junction 755) : after(0.9,sec)
  (junction 749) -> reset_return_arm_to_mag
  data: S_Inductive input; RQ_Delivery1 input; S_Part_Height input; RQ_Delivery2 input; ID_Delivery1 local; ID_Delivery2 local; S_Piston_Adv output; S_Elev_Down output; S_Pist_Fwd output; S_Part_Stuck output; S_Elev_Low output; S_Arm_Mag output; S_Arm_2_Mag output; S_Elev_High output; S_Suction_On output; S_Arm_2_Del output; S_Elev_Up output; S_Arm_Del output; S_Pist_Back output; S_Pist_Back_E output; S_Eject_Part output; S_Air_on output; S_S_Part output; S_On_d input; S_Suction_Off output; C_Start_d input; C_Manual input; C_Automatic input; C_Requested input; C_Identified input; S_Reset_d input; S_Part_Mag input; S_S_Station output; S_Off_t input; S_Key_Pos_t input; S_Panel_I4_t input; S_Panel_I5_t input; S_Panel_I6_t input; S_Led_Start_t output; S_Led_Reset_t output; S_Led_Extra2_t output; S_Panel_O7_t output; S_Led_Extra1_t output; S_Panel_O4_t output; S_Panel_O6_t output; S_Panel_O5_t output; S_Panel_I7_t input; S_On_t input; S_Off_d input; S_Key_Pos_d input; S_Panel_I6_d input; S_Panel_I5_d input; S_Panel_I7_d input; S_Panel_I4_d input; S_Panel_O6_d output; S_Led_Extra2_d output; S_Panel_O5_d output; S_Led_Start_d output; S_Led_Extra1_d output; S_Led_Reset_d output; S_Panel_O4_d output
